simulink model "controller_sg"  (R2022b)
settings: Solver=FixedStepAuto  StartTime=0.0  StopTime=100  FixedStep=0.005  RelTol=1e-3  EnableMultiTasking=on
undefined symbols (not defined in the file): MI_STATUSES, simp_vd_interface, simp_vd_lib
libraries: canmsglib x13, speedgoatlib_IO602_2_IO691 x5, battery_monitor_lib x1, driver_interface_lib x1, governor_lib x1, motor_interface_lib x1, simulink x1
settings Model: ExtModeTrigDuration=10  Creator=dr_pa  LastModifiedBy=maxfa
settings SolverCC: ConcurrentTasks=on  PositivePriorityOrder=on
settings DataIOCC: ExternalInput=Testbench_startup.getElement('AMK_bReserve'),Testbench_startup.getElement('DI_V_SteeringAngle'),Testbench_startup.getElement('DI_V_BrakePedalPos'),Testbench_startup.getElement('DI_b_DriverButton'),Testbench_startup.getElement('DI_V_AccelPedalPos1'),Testbench_startup.getElement('DI_V_AccelPedalPos2'),Testbench_startup.getElement('BM_b_prechrgContactorSts'),Testbench_startup.getElement('BM_b_HVposContactorSts'),Testbench_startup.getElement('BM_b_HVnegContactorSts'),Testbench_startup.getElement('AMK_bSystemReady'),Testbench_startup.getElement('AMK_bError'),Testbench_startup.getElement('AMK_bWarn'),Testbench_startup.getElement('AMK_bQuitDcOn'),Testbench_startup.getElement('AMK_bDcOn'),Testbench_startup.getElement('AMK_bQuitInverterOn'),Testbench_startup.getElement('AMK_bInverterOn'),Testbench_startup.getElement('AMK_bDerating'),Testbench_startup.getElement('AMK_TempMotor'),Testbench_startup.getElement('AMK_TempInverter'),Testbench_startup.getElement('AMK_ErrorInfo'),Testbench_startup.getElement('AMK_TempIGBT'),Testbench_startup.getElement('AMK_ActualVelocity'),Testbench_startup.getElement('AMK_TorqueCurrent'),Testbench_startup.getElement('AMK_MagnetizingCurrent')
settings OptimizationCC: BlockReduction=off  DefaultParameterBehavior=Inlined  OptimizeBlockIOStorage=off  EnhancedBackFolding=on  PassReuseOutputArgsThreshold=0  MaxStackSize=64  OptimizeBlockOrder=speed  DifferentSizesBufferReuse=on
settings DebuggingCC: TasksWithSamePriorityMsg=none  ParameterPrecisionLossMsg=none  ParameterTunabilityLossMsg=error
settings HardwareCC: ProdBitPerLong=64  ProdLongLongMode=on  ProdHWDeviceType=Intel->x86-64 (Linux 64)
settings SFSimCC: MATLABDynamicMemAlloc=off
settings RTWCC: Description=Simulink Real-Time  SystemTargetFile=slrealtime.tlc  TemplateMakefile=slrealtime_default_tmf  Toolchain=Simulink Real-Time Toolchain  BuildConfiguration=Faster Runs  CodeExecutionProfiling=on  TargetLang=C++
settings CodeAppCC: ForceParamTrailComments=on  OperatorAnnotations=on

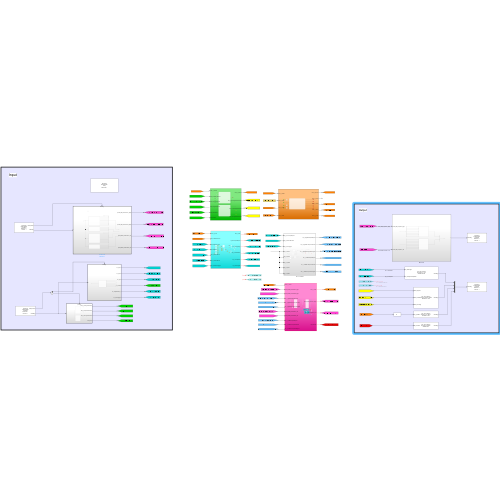
[thumbnail: Simulink's stored preview of the top-level diagram]
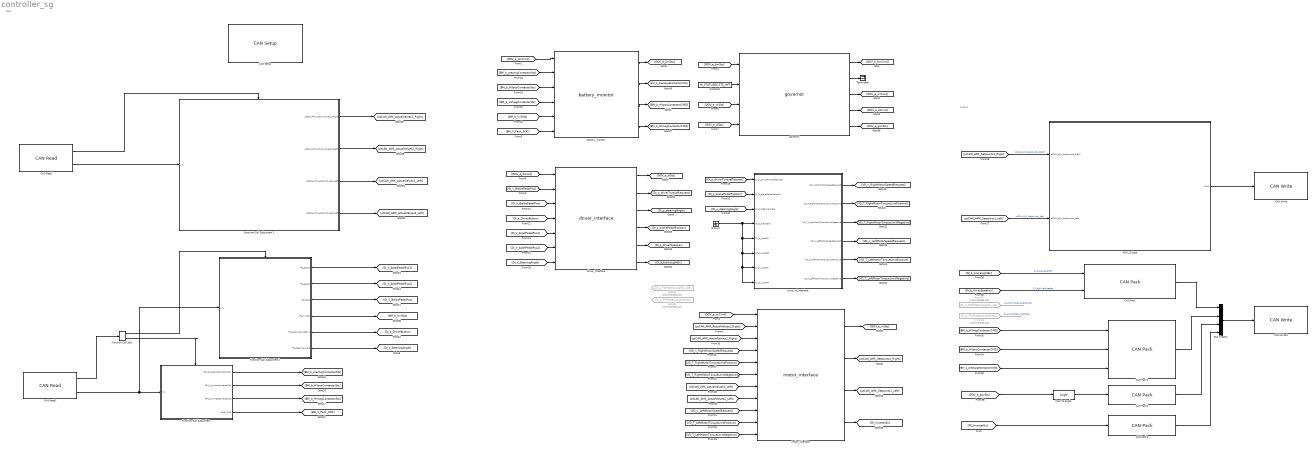
== system controller_sg ==
  note: Output
  note: Input
  AMK_Output : Subsystem
  Bus Creator : BusCreator  Inputs=4
  CAN Pack : canmsglib/CAN Pack  CANdbFile=C:\Users\maxfa\Documents\MAC FE\vehicle_control_system\src\VEH_CAN.dbc  MsgList=FC_cmd  MsgName=FC_cmd  MsgIDType=Standard (11-bit identifier)  MsgIdentifier=256  MsgLength=1  Remote=off  ApplyMinMax=off  BusOutput=off  SignalInfo={'FC_brakeLight','0','1','LE','unsigned','Standard','0','1','0','0','1';'FC_readyToDriveSpeaker','1','1','LE','unsigned','Standard','0','1','0','0','1'}
      settings: LibrarySourceBlock=embeddedtargetslib/Host Communication/CAN Pack  DataFormat=CANdb specified signals
  CAN Pack1 : canmsglib/CAN Pack  CANdbFile=C:\Users\maxfa\Documents\MAC FE\vehicle_control_system\src\VEH_CAN.dbc  MsgList=Contactor_States  MsgName=Contactor_States  MsgIDType=Standard (11-bit identifier)  MsgIdentifier=1570  MsgLength=3  Remote=off  ApplyMinMax=off  BusOutput=off  SignalInfo={'Pack_Negative','16','8','LE','unsigned','Standard','0','1','0','-Inf','Inf';'Pack_Positive','0','8','LE','unsigned','Standard','0','1','0','-Inf','Inf';'Pack_Precharge','8','8','LE','unsigned','Standard','0','1','0','-Inf','Inf'}
      settings: LibrarySourceBlock=embeddedtargetslib/Host Communication/CAN Pack  DataFormat=CANdb specified signals
  CAN Pack2 : canmsglib/CAN Pack  CANdbFile=C:\Users\maxfa\Documents\MAC FE\vehicle_control_system\src\VEH_CAN.dbc  MsgList=VC_Status  MsgName=VC_Status  MsgIDType=Standard (11-bit identifier)  MsgIdentifier=255  MsgLength=8  Remote=off  ApplyMinMax=off  BusOutput=off  SignalInfo={'VC_govStatus','0','3','LE','unsigned','Standard','0','1','0','0','7'}
      settings: LibrarySourceBlock=embeddedtargetslib/Host Communication/CAN Pack  DataFormat=CANdb specified signals
  CAN Pack3 : canmsglib/CAN Pack  CANdbFile=C:\Users\maxfa\Documents\MAC FE\can_dbc\dbcs\VEH_CAN.dbc  MsgList=InverterEn  MsgName=InverterEn  MsgIDType=Standard (11-bit identifier)  MsgIdentifier=0  MsgLength=1  Remote=off  ApplyMinMax=off  BusOutput=off  SignalInfo={'MI_InverterEn','0','1','LE','unsigned','Standard','0','1','0','0','1'}
      settings: LibrarySourceBlock=embeddedtargetslib/Host Communication/CAN Pack  DataFormat=CANdb specified signals
  CAN Read : speedgoatlib_IO602_2_IO691/CAN Read  id=1  ts=-1  channel=1  messageType=CAN  canType=CAN (HS)  BusOutput=off  initValues=[691 1 -1 0 1 1 0]
      settings: SourceProductName=Simulink Real-Time: Speedgoat I/O Blockset
  CAN Read1 : speedgoatlib_IO602_2_IO691/CAN Read  id=1  ts=-1  channel=1  messageType=CAN  canType=CAN (HS)  BusOutput=off  initValues=[691 1 -1 0 1 1 0]
      settings: SourceProductName=Simulink Real-Time: Speedgoat I/O Blockset
  "CAN Setup " : speedgoatlib_IO602_2_IO691/CAN Setup   moduletype=IO691  id=1  pciSlot=-1  chn1=CAN (HS)  chn2=Disabled  chn3=Disabled  chn4=Disabled  initStruct=[]  termStruct=[]  ArbitrationbdrChn1=500 kBaud  ArbitrationManbdrChn1=[2,16,63,16]  FdbdrChn1=5.0 MBaud  FdManbdrChn1=[2,2,5,2]  ArbitrationbdrChn2=1.0 MBaud  ArbitrationManbdrChn2=[2,8,31,8]  FdbdrChn2=5.0 MBaud  FdManbdrChn2=[2,2,5,2]  ArbitrationbdrChn3=1.0 MBaud  ArbitrationManbdrChn3=[2,8,31,8]  FdbdrChn3=5.0 MBaud  FdManbdrChn3=[2,2,5,2]  ArbitrationbdrChn4=1.0 MBaud  ArbitrationManbdrChn4=[2,8,31,8]  FdbdrChn4=5.0 MBaud  FdManbdrChn4=[2,2,5,2]  moduleInitValues=[691 1 -1 -1]
      settings: SourceProductName=Simulink Real-Time: Speedgoat I/O Blockset
  CAN Write : speedgoatlib_IO602_2_IO691/CAN Write  id=1  ts=-1  channel=1  messageType=CAN  BusInput=off  enableStatusPort=off  canType=CAN (HS)  initValues=[691 1 -1 0 1 1 0 0]
      settings: SourceProductName=Simulink Real-Time: Speedgoat I/O Blockset
  CAN Write1 : speedgoatlib_IO602_2_IO691/CAN Write  id=1  ts=-1  channel=1  messageType=CAN  BusInput=off  enableStatusPort=off  canType=CAN (HS)  initValues=[691 1 -1 0 1 1 0 0]
      settings: SourceProductName=Simulink Real-Time: Speedgoat I/O Blockset
  Cast To Single : DataTypeConversion  OutDataTypeStr=single  SaturateOnIntegerOverflow=off  RndMeth=Floor
  Constant : Constant  Value=MI_STATUSES.STS_INIT  OutDataTypeStr=Enum: MI_STATUSES
  From37 : From  Commented=on  GotoTag=DI_p_PWMstatusLightCycle
  From38 : From  Commented=on  GotoTag=DI_p_PWMstatusLightFreq
  Function-Call Split : FunctionCallSplit  IconShape=distinctive  NumOutputPorts=2  OutputPortLayout=default
  Function-Call Subsystem : Subsystem  TreatAsAtomicUnit=on
  Function-Call Subsystem1 : Subsystem  TreatAsAtomicUnit=on
  Function-Call Subsystem2 : Subsystem  TreatAsAtomicUnit=on
  Goto34 : Goto  Commented=on  GotoTag=DI_p_PWMstatusLightCycle
  Goto35 : Goto  Commented=on  GotoTag=DI_p_PWMstatusLightFreq
  Ground : Ground
  Terminator : Terminator
  battery_monitor : battery_monitor_lib/battery_monitor  SystemSampleTime=-1  VariantActivationTime=update diagram  Latency=0  AutoFrameSizeCalculation=off
  driver_interface : driver_interface_lib/driver_interface  SystemSampleTime=-1  VariantActivationTime=update diagram  Latency=0  AutoFrameSizeCalculation=off
  governor : governor_lib/governor  SystemSampleTime=-1  VariantActivationTime=update diagram  Latency=0  AutoFrameSizeCalculation=off
  motor_interface : motor_interface_lib/motor_interface  SystemSampleTime=-1  VariantActivationTime=update diagram  Latency=0  AutoFrameSizeCalculation=off
  simp_vd_interface : Subsystem  AncestorBlock=simp_vd_lib/simp_vd_interface
  wires:
  driver_interface/3 -> [DI_p_steeringAngle]
  driver_interface/5 -> [DI_b_driverSpeaker]
  [GOV_e_miSts] -> governor/3
  simp_vd_interface/6(VD_T_LeftMotorTorqueLimitNegative) -> [VD_T_LeftMotorTorqueLimitNegative]
  simp_vd_interface/4(VD_n_LeftMotorSpeedRequest) -> [VD_n_LeftMotorSpeedRequest]
  [VD_T_RightMotorTorqueLimitPositive] -> motor_interface/5
  driver_interface/4 -> [DI_p_brakePedalPosition]
  [DI_V_BrakePedalPos] -> driver_interface/2
  [ptCAN_AMK_Setpoints1_Left] -> AMK_Output/2(ptCAN_AMK_Setpoints1_Left)  "ptCAN_AMK_Setpoints1_Left"
  simp_vd_interface/3(VD_T_RightMotorTorqueLimitNegative) -> [VD_T_RightMotorTorqueLimitNegative]
  simp_vd_interface/1(VD_n_RightMotorSpeedRequest) -> [VD_n_RightMotorSpeedRequest]
  [DI_b_driverSpeaker] -> CAN Pack/2  "DI_b_driverSpeaker"
  [VD_T_RightMotorTorqueLimitNegative] -> motor_interface/6
  [DI_p_driverTorqueRequest] -> simp_vd_interface/1(DI_p_driverTorqueRequest)
  [DI_V_SteeringAngle] -> driver_interface/7
  [GOV_e_bmCmd] -> battery_monitor/1
  simp_vd_interface/2(VD_T_RightMotorTorqueLimitPositive) -> [VD_T_RightMotorTorqueLimitPositive]
  driver_interface/2 -> [DI_p_driverTorqueRequest]
  [DI_b_DriverButton] -> driver_interface/4
  [DI_V_AccelPedalPos1] -> driver_interface/5
  [DI_V_AccelPedalPos2] -> driver_interface/6
  driver_interface/1 -> [GOV_e_diSts]
  Constant/1 -> governor/2
  [ptCAN_AMK_ActualValues2_Right] -> motor_interface/3
  [GOV_e_bmSts] -> governor/1
  battery_monitor/1 -> [GOV_e_bmSts]
  [VD_n_RightMotorSpeedRequest] -> motor_interface/4
  simp_vd_interface/5(VD_T_LeftMotorTorqueLimitPositive) -> [VD_T_LeftMotorTorqueLimitPositive]
  governor/3 -> [GOV_e_miCmd]
  [GOV_e_diSts] -> governor/4
  [ptCAN_AMK_Setpoints1_Right] -> AMK_Output/1(ptCAN_AMK_Setpoints1_Right)  "ptCAN_AMK_Setpoints1_Right"
  [DI_V_BrakePedalPos] -> driver_interface/3
  [GOV_e_miCmd] -> motor_interface/1
  governor/4 -> [GOV_e_diCmd]
  [ptCAN_AMK_ActualValues1_Right] -> motor_interface/2
  governor/2 -> Terminator/1
  motor_interface/1 -> [GOV_e_miSts]
  [DI_p_brakePedalPosition] -> simp_vd_interface/2(DI_p_brakePedalPosition)
  governor/1 -> [GOV_e_bmCmd]
  motor_interface/2 -> [ptCAN_AMK_Setpoints1_Right]
  motor_interface/3 -> [ptCAN_AMK_Setpoints1_Left]
  [ptCAN_AMK_ActualValues1_Left] -> motor_interface/7
  [ptCAN_AMK_ActualValues2_Left] -> motor_interface/8
  [VD_n_LeftMotorSpeedRequest] -> motor_interface/9
  [VD_T_LeftMotorTorqueLimitPositive] -> motor_interface/10
  [VD_T_LeftMotorTorqueLimitNegative] -> motor_interface/11
  AMK_Output/1(Out1) -> CAN Write/1
  battery_monitor/2 -> [BM_b_prechargeContactorCMD]
  battery_monitor/4 -> [BM_b_HVnegContactorCMD]
  battery_monitor/3 -> [BM_b_HVposContactorCMD]
  driver_interface/6 -> [DI_b_brakeLightEn]
  [DI_b_brakeLightEn] -> CAN Pack/1  "DI_b_brakeLightEn"
  [DI_p_steeringAngle] -> simp_vd_interface/3(DI_p_steeringAngle)
  ? -> Goto34/1
  ? -> Goto35/1
  From37/1 -> ?  "DI_p_PWMstatusLightCycle"
  From38/1 -> ?  "DI_p_PWMstatusLightFreq"
  Function-Call Subsystem2/1(FC_apps1) -> [DI_V_AccelPedalPos1]
  Function-Call Subsystem2/2(FC_apps2) -> [DI_V_AccelPedalPos2]
  Function-Call Subsystem2/5(FC_ready2DriveBtn_n) -> [DI_b_DriverButton]
  Function-Call Subsystem2/3(FC_bpps) -> [DI_V_BrakePedalPos]
  CAN Pack/1 -> Bus Creator/1
  Function-Call Subsystem/1(BM_b_prechrgContactorSts) -> [BM_b_prechrgContactorSts]
  Function-Call Subsystem/2(BM_b_HVposContactorSts) -> [BM_b_HVposContactorSts]
  Function-Call Subsystem/3(BM_b_HVnegContactorSts) -> [BM_b_HVnegContactorSts]
  CAN Pack1/1 -> Bus Creator/2
  Bus Creator/1 -> CAN Write1/1
  CAN Read1/2 -> Function-Call Subsystem/1(In1), Function-Call Subsystem2/1(In1)
  Ground/1 -> simp_vd_interface/5(DI_p_wspdLR), simp_vd_interface/6(DI_p_wspdRR), simp_vd_interface/8(DI_p_wspdRF), simp_vd_interface/7(DI_p_wspdLF), simp_vd_interface/4(DI_b_tvEnable)
  governor/5 -> [GOV_e_govSts]
  CAN Pack2/1 -> Bus Creator/3
  [GOV_e_govSts] -> Cast To Single/1
  Cast To Single/1 -> CAN Pack2/1
  Function-Call Subsystem2/6(FC_steeringAngle) -> [DI_V_SteeringAngle]
  CAN Read/2 -> Function-Call Subsystem1/1(In1)
  Function-Call Subsystem1/1(ptCAN_AMK_ActualValues1_Right) -> [ptCAN_AMK_ActualValues1_Right]
  Function-Call Subsystem1/2(ptCAN_AMK_ActualValues2_Right) -> [ptCAN_AMK_ActualValues2_Right]
  Function-Call Subsystem1/3(ptCAN_AMK_ActualValues1_Left) -> [ptCAN_AMK_ActualValues1_Left]
  Function-Call Subsystem1/4(ptCAN_AMK_ActualValues2_Left) -> [ptCAN_AMK_ActualValues2_Left]
  Function-Call Split/2 -> Function-Call Subsystem/Trigger
  Function-Call Split/1 -> Function-Call Subsystem2/Trigger
  CAN Read1/1 -> Function-Call Split/1
  CAN Read/1 -> Function-Call Subsystem1/Trigger
  [GOV_e_diCmd] -> driver_interface/1
  [BM_b_prechrgContactorSts] -> battery_monitor/2
  [BM_b_HVposContactorSts] -> battery_monitor/3
  [BM_b_HVnegContactorSts] -> battery_monitor/4
  Function-Call Subsystem/4(Pack_SOC) -> [BM_V_Pack_SOC]
  [BM_V_Pack_SOC] -> battery_monitor/6
  Function-Call Subsystem2/4(FC_hvilSts) -> [BM_b_hvilSts]
  [BM_b_hvilSts] -> battery_monitor/5
  [BM_b_prechargeContactorCMD] -> CAN Pack1/3
  [BM_b_HVposContactorCMD] -> CAN Pack1/2
  [BM_b_HVnegContactorCMD] -> CAN Pack1/1
  CAN Pack3/1 -> Bus Creator/4
  motor_interface/4 -> [MI_InverterEn]
  [MI_InverterEn] -> CAN Pack3/1

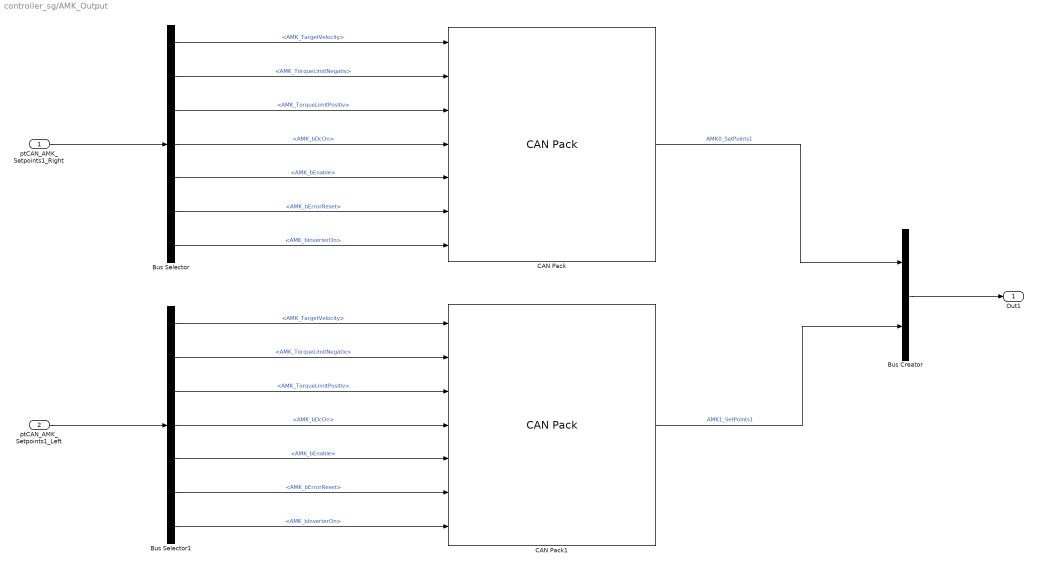
== system controller_sg/AMK_Output ==
  ptCAN_AMK_Setpoints1_Right : Inport
  ptCAN_AMK_Setpoints1_Left : Inport  Port=2
  Bus Creator : BusCreator  Inputs=2
  Bus Selector : BusSelector  OutputSignals=AMK_TargetVelocity,AMK_TorqueLimitNegativ,AMK_TorqueLimitPositiv,AMK_bDcOn,AMK_bEnable,AMK_bErrorReset,AMK_bInverterOn
  Bus Selector1 : BusSelector  OutputSignals=AMK_TargetVelocity,AMK_TorqueLimitNegativ,AMK_TorqueLimitPositiv,AMK_bDcOn,AMK_bEnable,AMK_bErrorReset,AMK_bInverterOn
  CAN Pack : canmsglib/CAN Pack  CANdbFile=C:\Users\LinF\Documents\MACFE\Embedded\CAN_Databases\CAN_AMKInverter.dbc  MsgList=AMK1_SetPoints1  MsgName=AMK1_SetPoints1  MsgIDType=Standard (11-bit identifier)  MsgIdentifier=390  MsgLength=8  Remote=off  ApplyMinMax=off  BusOutput=off  SignalInfo={'AMK_TargetVelocity','16','16','LE','signed','Standard','0','1','0','-Inf','Inf';'AMK_TorqueLimitNegativ','48','16','LE','signed','Standard','0','1','0','-Inf','Inf';'AMK_TorqueLimitPositiv','32','16','LE','signed','Standard','0','1','0','-Inf','Inf';'AMK_bDcOn','9','1','LE','unsigned','Standard','0','1','0','-Inf','Inf';'AMK_bEnable','10','1','LE','unsigned','Standard','0','1','0','-Inf','Inf';'AMK_bErrorReset','11','1','LE','unsigned','Standard','0','1','0','-Inf','Inf';'AMK_bInverterOn','8','1','LE','unsigned','Standard','0','1','0','-Inf','Inf'}
      settings: LibrarySourceBlock=canlib/CAN Pack  DataFormat=CANdb specified signals
  CAN Pack1 : canmsglib/CAN Pack  CANdbFile=C:\Users\LinF\Documents\MACFE\Embedded\CAN_Databases\CAN_AMKInverter.dbc  MsgList=AMK0_SetPoints1  MsgName=AMK0_SetPoints1  MsgIDType=Standard (11-bit identifier)  MsgIdentifier=389  MsgLength=8  Remote=off  ApplyMinMax=off  BusOutput=off  SignalInfo={'AMK_TargetVelocity','16','16','LE','signed','Standard','0','1','0','-Inf','Inf';'AMK_TorqueLimitNegativ','48','16','LE','signed','Standard','0','1','0','-Inf','Inf';'AMK_TorqueLimitPositiv','32','16','LE','signed','Standard','0','1','0','-Inf','Inf';'AMK_bDcOn','9','1','LE','unsigned','Standard','0','1','0','-Inf','Inf';'AMK_bEnable','10','1','LE','unsigned','Standard','0','1','0','-Inf','Inf';'AMK_bErrorReset','11','1','LE','unsigned','Standard','0','1','0','-Inf','Inf';'AMK_bInverterOn','8','1','LE','unsigned','Standard','0','1','0','-Inf','Inf'}
      settings: LibrarySourceBlock=canlib/CAN Pack  DataFormat=CANdb specified signals
  Out1 : Outport
  wires:
  CAN Pack/1 -> Bus Creator/1  "AMK0_SetPoints1"
  CAN Pack1/1 -> Bus Creator/2  "AMK1_SetPoints1"
  Bus Selector/7 -> CAN Pack/7  "<AMK_bInverterOn>"
  Bus Selector/4 -> CAN Pack/4  "<AMK_bDcOn>"
  Bus Selector/5 -> CAN Pack/5  "<AMK_bEnable>"
  Bus Selector/6 -> CAN Pack/6  "<AMK_bErrorReset>"
  Bus Selector/1 -> CAN Pack/1  "<AMK_TargetVelocity>"
  Bus Selector/3 -> CAN Pack/3  "<AMK_TorqueLimitPositiv>"
  Bus Selector/2 -> CAN Pack/2  "<AMK_TorqueLimitNegativ>"
  Bus Creator/1 -> Out1/1
  Bus Selector1/1 -> CAN Pack1/1  "<AMK_TargetVelocity>"
  Bus Selector1/3 -> CAN Pack1/3  "<AMK_TorqueLimitPositiv>"
  Bus Selector1/2 -> CAN Pack1/2  "<AMK_TorqueLimitNegativ>"
  Bus Selector1/4 -> CAN Pack1/4  "<AMK_bDcOn>"
  Bus Selector1/5 -> CAN Pack1/5  "<AMK_bEnable>"
  Bus Selector1/6 -> CAN Pack1/6  "<AMK_bErrorReset>"
  Bus Selector1/7 -> CAN Pack1/7  "<AMK_bInverterOn>"
  ptCAN_AMK_Setpoints1_Right/1 -> Bus Selector/1
  ptCAN_AMK_Setpoints1_Left/1 -> Bus Selector1/1

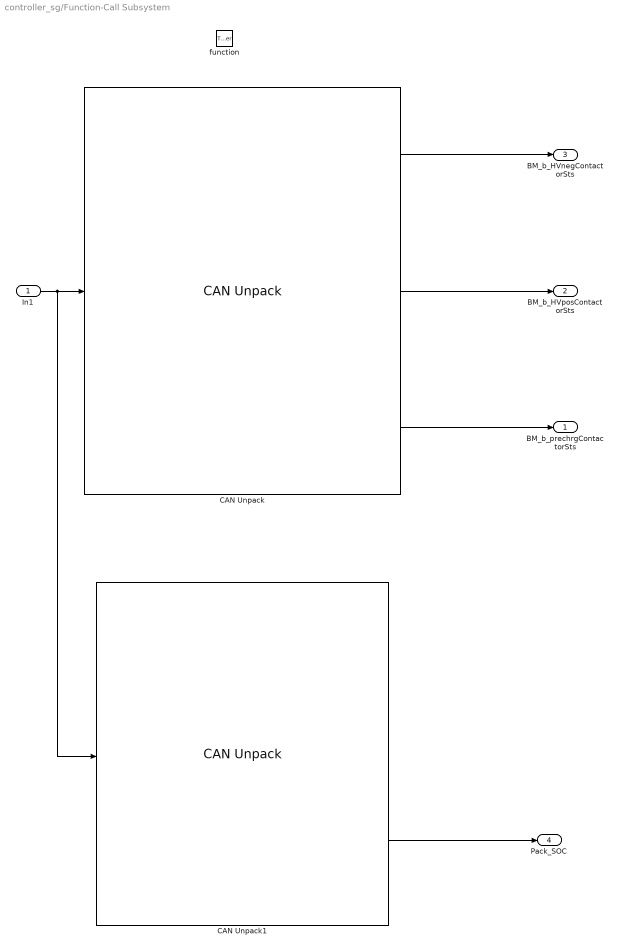
== system controller_sg/Function-Call Subsystem ==
  In1 : Inport
  function : TriggerPort  TriggerType=function-call  VariantControl=(inherit)
  CAN Unpack : canmsglib/CAN Unpack  CANdbFile=C:\Users\LinF\Documents\MACFE\Controls\repos\can_dbc\dbcs\VEH_CAN.dbc  MsgList=Contactor_Feedback  MsgName=Contactor_Feedback  MsgIDType=Standard (11-bit identifier)  MsgIdentifier=1574  MsgLength=3  SignalInfo={'Pack_Negative_Feedback','8','1','LE','unsigned','Standard','0','1','0','0','1';'Pack_Positive_Feedback','0','1','LE','unsigned','Standard','0','1','0','0','1';'Pack_Precharge_Feedback','16','1','LE','unsigned','Standard','0','1','0','0','1'}  IDPort=off  TimestampPort=off  ErrorPort=off  RemotePort=off  LengthPort=off  StatusPort=off  ApplyMinMax=off
      settings: LibrarySourceBlock=canlib/CAN Unpack  DataFormat=CANdb specified signals
  CAN Unpack1 : canmsglib/CAN Unpack  CANdbFile=C:\Users\maxfa\Documents\MAC FE\vehicle_control_system\src\VEH_CAN.dbc  MsgList=Pack_SOC  MsgName=Pack_SOC  MsgIDType=Standard (11-bit identifier)  MsgIdentifier=1573  MsgLength=3  SignalInfo={'Maximum_Pack_Voltage','8','16','LE','unsigned','Standard','0','0.1','0','-Inf','Inf';'Pack_SOC','0','8','LE','unsigned','Standard','0','0.5','0','-Inf','Inf'}  IDPort=off  TimestampPort=off  ErrorPort=off  RemotePort=off  LengthPort=off  StatusPort=off  ApplyMinMax=off
      settings: LibrarySourceBlock=embeddedtargetslib/Host Communication/CAN Unpack  DataFormat=CANdb specified signals
  BM_b_prechrgContactorSts : Outport
  BM_b_HVposContactorSts : Outport  Port=2
  BM_b_HVnegContactorSts : Outport  Port=3
  Pack_SOC : Outport  Port=4
  wires:
  CAN Unpack/1 -> BM_b_HVnegContactorSts/1
  CAN Unpack/2 -> BM_b_HVposContactorSts/1
  In1/1 -> CAN Unpack1/1, CAN Unpack/1
  CAN Unpack/3 -> BM_b_prechrgContactorSts/1
  CAN Unpack1/2 -> Pack_SOC/1

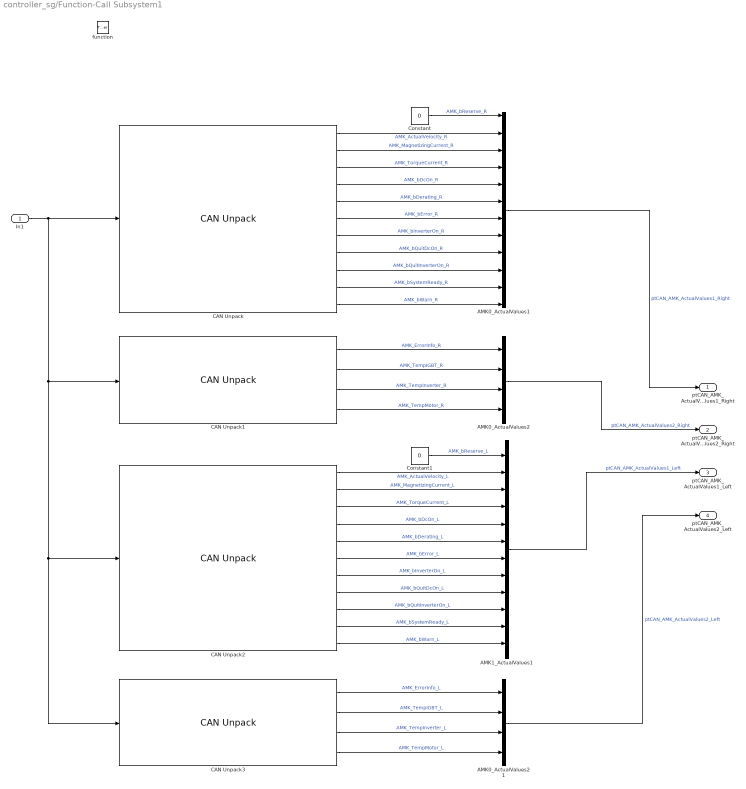
== system controller_sg/Function-Call Subsystem1 ==
  In1 : Inport
  function : TriggerPort  TriggerType=function-call  VariantControl=(inherit)
  "AMK0_ActualValues1 " : BusCreator  Inputs=12
  "AMK0_ActualValues2 " : BusCreator  Inputs=4
  AMK0_ActualValues2 1 : BusCreator  Inputs=4
  AMK1_ActualValues1 : BusCreator  Inputs=12
  CAN Unpack : canmsglib/CAN Unpack  CANdbFile=C:\Users\LinF\Documents\MACFE\Embedded\CAN_Stuff\CAN_Databases\CAN_AMKInverter.dbc  MsgList=AMK1_ActualValues1  MsgName=AMK1_ActualValues1  MsgIDType=Standard (11-bit identifier)  MsgIdentifier=645  MsgLength=8  SignalInfo={'AMK_ActualVelocity','16','16','LE','signed','Standard','0','1','0','-Inf','Inf';'AMK_MagnetizingCurrent','48','16','LE','signed','Standard','0','1','0','-Inf','Inf';'AMK_TorqueCurrent','32','16','LE','signed','Standard','0','1','0','-Inf','Inf';'AMK_bDcOn','12','1','LE','unsigned','Standard','0','1','0','-Inf','Inf';'AMK_bDerating','15','1','LE','unsigned','Standard','0','1','0','-Inf','Inf';'AMK_bError','9','1','LE','unsigned','Standard','0','1','0','-Inf','Inf';'AMK_bInverterOn','14','1','LE','unsigned','Standard','0','1','0','-Inf','Inf';'AMK_bQuitDcOn','11','1','LE','unsigned','Standard','0','1','0','-Inf','Inf';'AMK_bQuitInverterOn','13','1','LE','unsigned','Standard','0','1','0','-Inf','Inf';'AMK_bSystemReady','8','1','LE','unsigned','Standard','0','1','0','-Inf','Inf';'AMK_bWarn','10','1','LE','unsigned','Standard','0','1','0','-Inf','Inf'}  IDPort=off  TimestampPort=off  ErrorPort=off  RemotePort=off  LengthPort=off  StatusPort=off  ApplyMinMax=off
      settings: LibrarySourceBlock=canlib/CAN Unpack  DataFormat=CANdb specified signals
  CAN Unpack1 : canmsglib/CAN Unpack  CANdbFile=C:\Users\LinF\Documents\MACFE\Embedded\CAN_Stuff\CAN_Databases\CAN_AMKInverter.dbc  MsgList=AMK1_ActualValues2  MsgName=AMK1_ActualValues2  MsgIDType=Standard (11-bit identifier)  MsgIdentifier=647  MsgLength=8  SignalInfo={'AMK_ErrorInfo','32','16','LE','unsigned','Standard','0','1','0','0','65535';'AMK_TempIGBT','48','16','LE','signed','Standard','0','0.1','0','-3276.8','3276.7';'AMK_TempInverter','16','16','LE','signed','Standard','0','0.1','0','-3276.8','3276.7';'AMK_TempMotor','0','16','LE','signed','Standard','0','0.1','0','-3276.8','3276.7'}  IDPort=off  TimestampPort=off  ErrorPort=off  RemotePort=off  LengthPort=off  StatusPort=off  ApplyMinMax=off
      settings: LibrarySourceBlock=canlib/CAN Unpack  DataFormat=CANdb specified signals
  CAN Unpack2 : canmsglib/CAN Unpack  CANdbFile=C:\Users\LinF\Documents\MACFE\Embedded\CAN_Stuff\CAN_Databases\CAN_AMKInverter.dbc  MsgList=AMK0_ActualValues1  MsgName=AMK0_ActualValues1  MsgIDType=Standard (11-bit identifier)  MsgIdentifier=644  MsgLength=8  SignalInfo={'AMK_ActualVelocity','16','16','LE','signed','Standard','0','1','0','-Inf','Inf';'AMK_MagnetizingCurrent','48','16','LE','signed','Standard','0','1','0','-Inf','Inf';'AMK_TorqueCurrent','32','16','LE','signed','Standard','0','1','0','-Inf','Inf';'AMK_bDcOn','12','1','LE','unsigned','Standard','0','1','0','-Inf','Inf';'AMK_bDerating','15','1','LE','unsigned','Standard','0','1','0','-Inf','Inf';'AMK_bError','9','1','LE','unsigned','Standard','0','1','0','-Inf','Inf';'AMK_bInverterOn','14','1','LE','unsigned','Standard','0','1','0','-Inf','Inf';'AMK_bQuitDcOn','11','1','LE','unsigned','Standard','0','1','0','-Inf','Inf';'AMK_bQuitInverterOn','13','1','LE','unsigned','Standard','0','1','0','-Inf','Inf';'AMK_bSystemReady','8','1','LE','unsigned','Standard','0','1','0','-Inf','Inf';'AMK_bWarn','10','1','LE','unsigned','Standard','0','1','0','-Inf','Inf'}  IDPort=off  TimestampPort=off  ErrorPort=off  RemotePort=off  LengthPort=off  StatusPort=off  ApplyMinMax=off
      settings: LibrarySourceBlock=canlib/CAN Unpack  DataFormat=CANdb specified signals
  CAN Unpack3 : canmsglib/CAN Unpack  CANdbFile=C:\Users\LinF\Documents\MACFE\Embedded\CAN_Stuff\CAN_Databases\CAN_AMKInverter.dbc  MsgList=AMK0_ActualValues2  MsgName=AMK0_ActualValues2  MsgIDType=Standard (11-bit identifier)  MsgIdentifier=646  MsgLength=8  SignalInfo={'AMK_ErrorInfo','32','16','LE','unsigned','Standard','0','1','0','0','65535';'AMK_TempIGBT','48','16','LE','signed','Standard','0','0.1','0','-3276.8','3276.7';'AMK_TempInverter','16','16','LE','signed','Standard','0','0.1','0','-3276.8','3276.7';'AMK_TempMotor','0','16','LE','signed','Standard','0','0.1','0','-3276.8','3276.7'}  IDPort=off  TimestampPort=off  ErrorPort=off  RemotePort=off  LengthPort=off  StatusPort=off  ApplyMinMax=off
      settings: LibrarySourceBlock=canlib/CAN Unpack  DataFormat=CANdb specified signals
  Constant : Constant  Value=0
  Constant1 : Constant  Value=0
  ptCAN_AMK_ActualValues1_Right : Outport
  ptCAN_AMK_ActualValues2_Right : Outport  Port=2
  ptCAN_AMK_ActualValues1_Left : Outport  Port=3
  ptCAN_AMK_ActualValues2_Left : Outport  Port=4
  wires:
  CAN Unpack3/4 -> AMK0_ActualValues2 1/4  "AMK_TempMotor_L"
  Constant/1 -> "AMK0_ActualValues1 "/1  "AMK_bReserve_R"
  CAN Unpack2/11 -> AMK1_ActualValues1/12  "AMK_bWarn_L"
  CAN Unpack2/9 -> AMK1_ActualValues1/10  "AMK_bQuitInverterOn_L"
  Constant1/1 -> AMK1_ActualValues1/1  "AMK_bReserve_L"
  CAN Unpack2/6 -> AMK1_ActualValues1/7  "AMK_bError_L"
  CAN Unpack3/3 -> AMK0_ActualValues2 1/3  "AMK_TempInverter_L"
  AMK1_ActualValues1/1 -> ptCAN_AMK_ActualValues1_Left/1  "ptCAN_AMK_ActualValues1_Left"
  CAN Unpack1/4 -> "AMK0_ActualValues2 "/4  "AMK_TempMotor_R"
  AMK0_ActualValues2 1/1 -> ptCAN_AMK_ActualValues2_Left/1  "ptCAN_AMK_ActualValues2_Left"
  CAN Unpack2/8 -> AMK1_ActualValues1/9  "AMK_bQuitDcOn_L"
  CAN Unpack3/1 -> AMK0_ActualValues2 1/1  "AMK_ErrorInfo_L"
  CAN Unpack2/5 -> AMK1_ActualValues1/6  "AMK_bDerating_L"
  CAN Unpack/7 -> "AMK0_ActualValues1 "/8  "AMK_bInverterOn_R"
  CAN Unpack2/10 -> AMK1_ActualValues1/11  "AMK_bSystemReady_L"
  CAN Unpack/6 -> "AMK0_ActualValues1 "/7  "AMK_bError_R"
  CAN Unpack/11 -> "AMK0_ActualValues1 "/12  "AMK_bWarn_R"
  CAN Unpack/2 -> "AMK0_ActualValues1 "/3  "AMK_MagnetizingCurrent_R"
  CAN Unpack1/2 -> "AMK0_ActualValues2 "/2  "AMK_TempIGBT_R"
  CAN Unpack/5 -> "AMK0_ActualValues1 "/6  "AMK_bDerating_R"
  "AMK0_ActualValues1 "/1 -> ptCAN_AMK_ActualValues1_Right/1  "ptCAN_AMK_ActualValues1_Right"
  CAN Unpack/8 -> "AMK0_ActualValues1 "/9  "AMK_bQuitDcOn_R"
  CAN Unpack2/2 -> AMK1_ActualValues1/3  "AMK_MagnetizingCurrent_L"
  CAN Unpack1/1 -> "AMK0_ActualValues2 "/1  "AMK_ErrorInfo_R"
  CAN Unpack2/4 -> AMK1_ActualValues1/5  "AMK_bDcOn_L"
  CAN Unpack2/1 -> AMK1_ActualValues1/2  "AMK_ActualVelocity_L"
  CAN Unpack/10 -> "AMK0_ActualValues1 "/11  "AMK_bSystemReady_R"
  CAN Unpack/9 -> "AMK0_ActualValues1 "/10  "AMK_bQuitInverterOn_R"
  CAN Unpack/4 -> "AMK0_ActualValues1 "/5  "AMK_bDcOn_R"
  CAN Unpack2/7 -> AMK1_ActualValues1/8  "AMK_bInverterOn_L"
  In1/1 -> CAN Unpack3/1, CAN Unpack2/1, CAN Unpack1/1, CAN Unpack/1
  CAN Unpack/3 -> "AMK0_ActualValues1 "/4  "AMK_TorqueCurrent_R"
  "AMK0_ActualValues2 "/1 -> ptCAN_AMK_ActualValues2_Right/1  "ptCAN_AMK_ActualValues2_Right"
  CAN Unpack2/3 -> AMK1_ActualValues1/4  "AMK_TorqueCurrent_L"
  CAN Unpack3/2 -> AMK0_ActualValues2 1/2  "AMK_TempIGBT_L"
  CAN Unpack/1 -> "AMK0_ActualValues1 "/2  "AMK_ActualVelocity_R"
  CAN Unpack1/3 -> "AMK0_ActualValues2 "/3  "AMK_TempInverter_R"

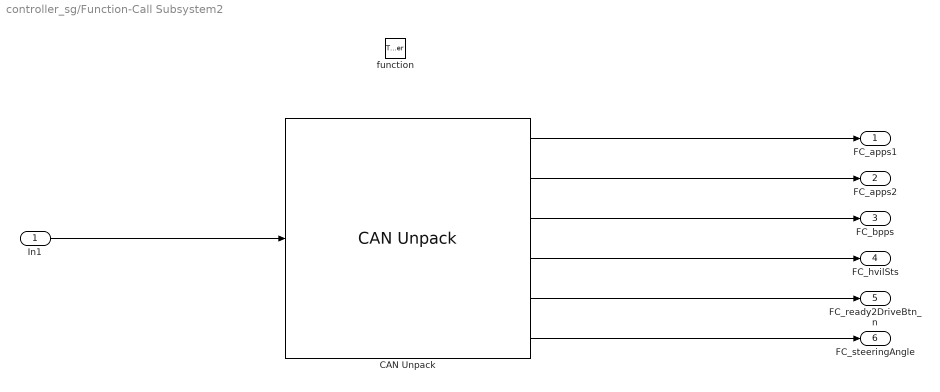
== system controller_sg/Function-Call Subsystem2 ==
  In1 : Inport
  function : TriggerPort  TriggerType=function-call  VariantControl=(inherit)
  CAN Unpack : canmsglib/CAN Unpack  CANdbFile=C:\Users\LinF\Documents\MACFE\Controls\repos\can_dbc\dbcs\VEH_CAN.dbc  MsgList=FC_msg  MsgName=FC_msg  MsgIDType=Standard (11-bit identifier)  MsgIdentifier=511  MsgLength=8  SignalInfo={'FC_apps1','0','12','LE','unsigned','Standard','0','1','0','0','4095';'FC_apps2','16','12','LE','unsigned','Standard','0','1','0','0','4095';'FC_bpps','32','12','LE','unsigned','Standard','0','1','0','0','4095';'FC_hvilSts','60','1','LE','unsigned','Standard','0','1','0','0','1';'FC_readyToDriveBtn_n','61','1','LE','unsigned','Standard','0','1','0','0','1';'FC_steeringAngle','48','12','LE','unsigned','Standard','0','1','0','0','4095'}  IDPort=off  TimestampPort=off  ErrorPort=off  RemotePort=off  LengthPort=off  StatusPort=off  ApplyMinMax=off
      settings: LibrarySourceBlock=canlib/CAN Unpack  DataFormat=CANdb specified signals
  FC_apps1 : Outport
  FC_apps2 : Outport  Port=2
  FC_bpps : Outport  Port=3
  FC_hvilSts : Outport  Port=4
  FC_ready2DriveBtn_n : Outport  Port=5
  FC_steeringAngle : Outport  Port=6
  wires:
  CAN Unpack/6 -> FC_steeringAngle/1
  CAN Unpack/5 -> FC_ready2DriveBtn_n/1
  CAN Unpack/2 -> FC_apps2/1
  CAN Unpack/3 -> FC_bpps/1
  CAN Unpack/1 -> FC_apps1/1
  In1/1 -> CAN Unpack/1
  CAN Unpack/4 -> FC_hvilSts/1

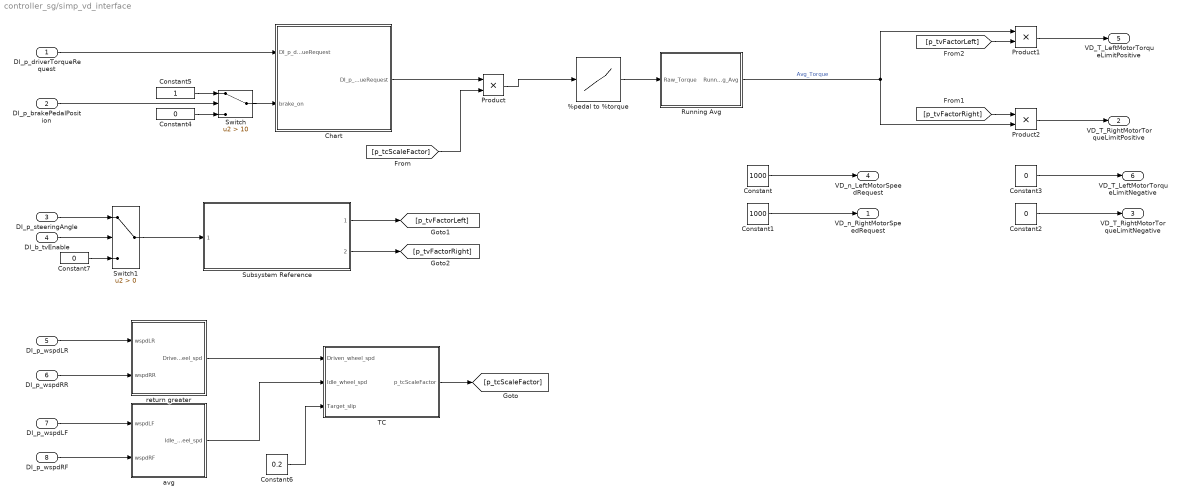
== system controller_sg/simp_vd_interface ==
  DI_p_driverTorqueRequest : Inport
  DI_p_brakePedalPosition : Inport  Port=2
  DI_p_steeringAngle : Inport  Port=3
  DI_b_tvEnable : Inport  Port=4
  DI_p_wspdLR : Inport  Port=5
  DI_p_wspdRR : Inport  Port=6
  DI_p_wspdLF : Inport  Port=7
  DI_p_wspdRF : Inport  Port=8
  %pedal to %torque : Lookup_n-D  NumberOfTableDimensions=1  BreakpointsForDimension1=[linspace(0,100,101)]  Table=[linspace(0,1000,101)]  InternalRulePriority=Speed  RndMeth=Simplest
  Chart : Stateflow chart  TreatAsAtomicUnit=on
  Constant : Constant  Value=1000
  Constant1 : Constant  Value=1000
  Constant{2..4,7} (4 alike) : Constant  Value=0
  Constant5 : Constant
  Constant6 : Constant  Value=0.2
  Product : Product
  Product1 : Product
  Product2 : Product
  Running Avg : Subsystem
  Subsystem Reference : Subsystem  ReferencedSubsystem=open_loop_tv
  Switch : Switch  Criteria=u2 > Threshold  Threshold=10  SaturateOnIntegerOverflow=off  InputSameDT=off
  Switch1 : Switch  Criteria=u2 > Threshold  SaturateOnIntegerOverflow=off  InputSameDT=off
  TC : Subsystem
  avg : MATLAB Function  TreatAsAtomicUnit=on
  return greater : MATLAB Function  TreatAsAtomicUnit=on
  VD_n_RightMotorSpeedRequest : Outport
  VD_T_RightMotorTorqueLimitPositive : Outport  Port=2
  VD_T_RightMotorTorqueLimitNegative : Outport  Port=3
  VD_n_LeftMotorSpeedRequest : Outport  Port=4
  VD_T_LeftMotorTorqueLimitPositive : Outport  Port=5
  VD_T_LeftMotorTorqueLimitNegative : Outport  Port=6
  wires:
  [p_tcScaleFactor] -> Product/2
  TC/1(p_tcScaleFactor) -> [p_tcScaleFactor]
  Product/1 -> %pedal to %torque/1
  Constant6/1 -> TC/3(Target_slip)
  return greater/1(Driven_wheel_spd) -> TC/1(Driven_wheel_spd)
  DI_p_wspdRR/1 -> return greater/2(wspdRR)
  DI_p_wspdLR/1 -> return greater/1(wspdLR)
  avg/1(Idle_wheel_spd) -> TC/2(Idle_wheel_spd)
  DI_p_wspdRF/1 -> avg/2(wspdRF)
  DI_p_wspdLF/1 -> avg/1(wspdLF)
  DI_p_steeringAngle/1 -> Switch1/1
  Constant/1 -> VD_n_LeftMotorSpeedRequest/1
  Constant1/1 -> VD_n_RightMotorSpeedRequest/1
  Constant2/1 -> VD_T_RightMotorTorqueLimitNegative/1
  Constant3/1 -> VD_T_LeftMotorTorqueLimitNegative/1
  Constant4/1 -> Switch/3
  Constant5/1 -> Switch/1
  Switch/1 -> Chart/2(brake_on)
  DI_p_brakePedalPosition/1 -> Switch/2
  DI_p_driverTorqueRequest/1 -> Chart/1(DI_p_driverTorqueRequest)
  %pedal to %torque/1 -> Running Avg/1(Raw_Torque)
  Running Avg/1(Running_Avg) -> Product2/2, Product1/1  "Avg_Torque"
  Chart/1(DI_p_motorTorqueRequest) -> Product/1
  Subsystem Reference/1 -> [p_tvFactorLeft]
  Subsystem Reference/2 -> [p_tvFactorRight]
  Product1/1 -> VD_T_LeftMotorTorqueLimitPositive/1
  Product2/1 -> VD_T_RightMotorTorqueLimitPositive/1
  [p_tvFactorRight] -> Product2/1
  [p_tvFactorLeft] -> Product1/2
  Switch1/1 -> Subsystem Reference/1
  DI_b_tvEnable/1 -> Switch1/2
  Constant7/1 -> Switch1/3

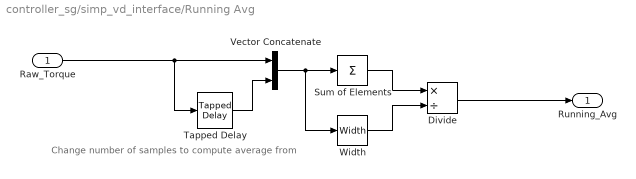
== system controller_sg/simp_vd_interface/Running Avg ==
  note: Change number of samples to compute average from
  Raw_Torque : Inport
  Divide : Product  Inputs=*/
  Sum of Elements : Sum  Inputs=+
  Tapped Delay : simulink/Discrete/Tapped Delay  vinit=0  samptime=-1  NumDelays=10  DelayOrder=Oldest  includeCurrent=off
  Vector Concatenate : Concatenate
  Width : Width
  Running_Avg : Outport
  wires:
  Divide/1 -> Running_Avg/1
  Vector Concatenate/1 -> Width/1, Sum of Elements/1
  Raw_Torque/1 -> Vector Concatenate/1, Tapped Delay/1
  Width/1 -> Divide/2
  Tapped Delay/1 -> Vector Concatenate/2
  Sum of Elements/1 -> Divide/1

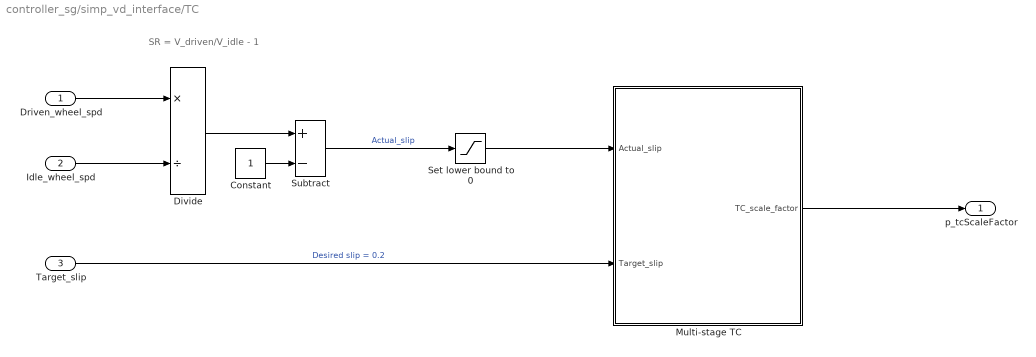
== system controller_sg/simp_vd_interface/TC ==
  note: SR = V_driven/V_idle - 1
  Driven_wheel_spd : Inport
  Idle_wheel_spd : Inport  Port=2
  Target_slip : Inport  Port=3
  Constant : Constant
  Divide : Product  Inputs=*/
  Multi-stage TC : Stateflow chart  TreatAsAtomicUnit=on
  Set lower bound to 0 : Saturate  UpperLimit=inf  LowerLimit=0
  Subtract : Sum  Inputs=+-
  p_tcScaleFactor : Outport
  wires:
  Set lower bound to 0/1 -> Multi-stage TC/1(Actual_slip)
  Constant/1 -> Subtract/2
  Divide/1 -> Subtract/1
  Driven_wheel_spd/1 -> Divide/1
  Idle_wheel_spd/1 -> Divide/2
  Target_slip/1 -> Multi-stage TC/2(Target_slip)  "Desired slip = 0.2"
  Subtract/1 -> Set lower bound to 0/1  "Actual_slip"
  Multi-stage TC/1(TC_scale_factor) -> p_tcScaleFactor/1

== stateflow chart controller_sg/simp_vd_interface/TC/Multi-stage TC ==
  state TC_off
    en, du:
    TC_scale_factor = 1;
  state TC_on
    en, du:
    TC_scale_factor = 0.5;
  state TC_on1
    en, du:
    TC_scale_factor = 0.25;
  state TC_on2
    en, du:
    TC_scale_factor = 0;
  (default) -> TC_off
  TC_off -> TC_on2 : [after(50,msec) && Actual_slip > Target_slip]
  TC_on -> TC_off : after(33,msec)
  TC_on1 -> TC_on : after(33,msec)
  TC_on2 -> TC_on1 : [after(33,msec) && Actual_slip <= Target_slip]
  data: Actual_slip input; Target_slip input; TC_scale_factor output

== matlab function controller_sg/simp_vd_interface/avg ==
  data: wspdLF input; Idle_wheel_spd output; wspdRF input
function Idle_wheel_spd = fcn(wspdLF,wspdRF)
Idle_wheel_spd = (wspdLF+wspdRF)/2;

== stateflow chart controller_sg/simp_vd_interface/Chart ==
  state Run
    en, du:
    DI_p_motorTorqueRequest = DI_p_driverTorqueRequest;
  state Stop
    en, du:
    DI_p_motorTorqueRequest = 0;
  (default) -> Run
  Run -> Stop : [DI_p_driverTorqueRequest >= 25 && brake_on]
  Stop -> Run : [DI_p_driverTorqueRequest < 5 && ~brake_on]
  data: DI_p_driverTorqueRequest input; brake_on input; DI_p_motorTorqueRequest output

== matlab function controller_sg/simp_vd_interface/return greater ==
  data: wspdLR input; Driven_wheel_spd output; wspdRR input
function Driven_wheel_spd = fcn(wspdLR,wspdRR)
if wspdLR > wspdRR
    Driven_wheel_spd = wspdLR;
else
    Driven_wheel_spd = wspdRR;
end
